simulink model "Plant"  (R2015b)
settings: Solver=ode45  StartTime=0.0  StopTime=1200  RelTol=1e-3
libraries: simulink x2, aerolibanimutils x1
settings Model: Creator=jruesch  LastModifiedBy=jruesch
settings DataIOCC: MaxDataPoints=1  SaveFinalState=on  SaveCompleteFinalSimState=on  SaveFormat=Array  SaveOutput=off  SignalLogging=off  DSMLogging=off  VisualizeSimOutput=off  SaveTime=off
settings HardwareCC: ProdBitPerPointer=32  ProdLargestAtomicFloat=None  ProdIntDivRoundTo=Undefined  ProdEndianess=Unspecified  ProdWordSize=32  ProdHWDeviceType=32-bit Generic
settings GRTTargetCC: GeneratePreprocessorConditionals=Disable all
settings ConfigComp: CovModelRefEnable=Off

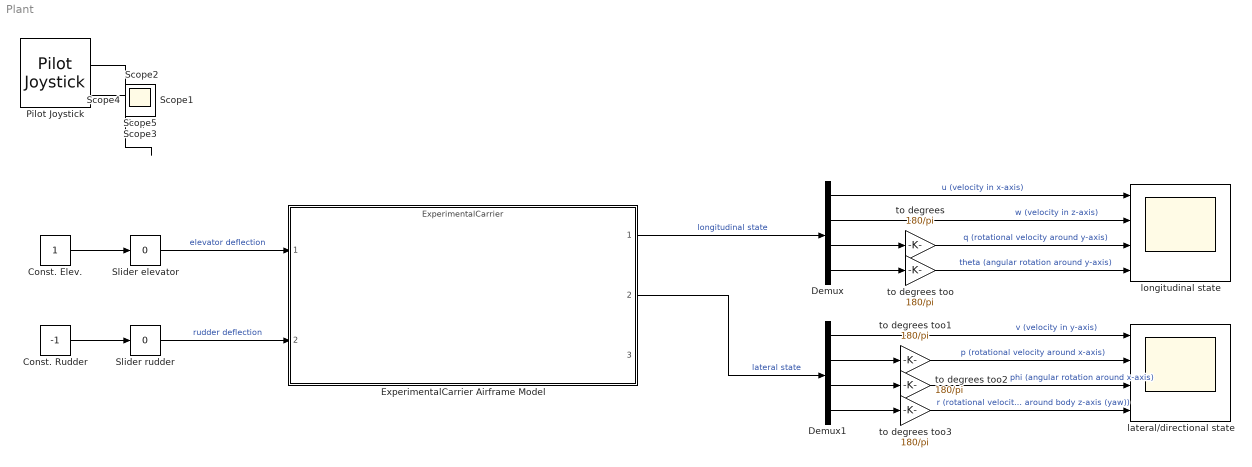
== system Plant ==
  Const. Elev. : Constant
  Const. Rudder : Constant  Value=-1
  Demux : Demux
  Demux1 : Demux
  ExperimentalCarrier Airframe Model : ModelReference  ModelNameDialog=ExperimentalCarrier.slx  SimulationMode=Normal  ModelReferenceVersion=1.534  CopyOfModelName=ExperimentalCarrier.slx
      mask Display: image(imread('../../figures/Airframe01.png'))
  Pilot Joystick : aerolibanimutils/Pilot Joystick  JoystickID=None  OutputConfiguration=FourAxis  SampleTime=1/30
  Slider rudder : simulink/Math Operations/Slider Gain  low=-0.2  gain=0  high=0.2
  Slider elevator : simulink/Math Operations/Slider Gain  low=-0.2  gain=0  high=0.2
  lateral/directional state : Scope  NumInputPorts=4
  longitudinal state : Scope  NumInputPorts=4
  to degrees : Gain  Gain=180/pi
  to degrees too{,1..3} (4 alike) : Gain  Gain=180/pi
  Scope{,1..5} (6 alike) : Scope
  wires:
  Pilot Joystick/4 -> ?
  Pilot Joystick/2 -> ?
  Slider rudder/1 -> ExperimentalCarrier Airframe Model/2  "rudder deflection"
  Slider elevator/1 -> ExperimentalCarrier Airframe Model/1  "elevator deflection"
  ExperimentalCarrier Airframe Model/1 -> Demux/1  "longitudinal state"
  ExperimentalCarrier Airframe Model/2 -> Demux1/1  "lateral state"
  Demux/1 -> longitudinal state/1  "u (velocity in x-axis)"
  Demux/2 -> longitudinal state/2  "w (velocity in z-axis)"
  Demux/3 -> to degrees/1
  Demux/4 -> to degrees too/1
  Demux1/1 -> lateral/directional state/1  "v (velocity in y-axis)"
  Demux1/2 -> to degrees too1/1
  Demux1/3 -> to degrees too2/1
  Demux1/4 -> to degrees too3/1
  to degrees/1 -> longitudinal state/3  "q (rotational velocity around y-axis)"
  to degrees too/1 -> longitudinal state/4  "theta (angular rotation around y-axis)"
  to degrees too1/1 -> lateral/directional state/2  "p (rotational velocity around x-axis)"
  to degrees too2/1 -> lateral/directional state/3  "phi (angular rotation around x-axis)"
  to degrees too3/1 -> lateral/directional state/4  "r (rotational velocity around body z-axis (yaw))"
  Const. Elev./1 -> Slider elevator/1
  Const. Rudder/1 -> Slider rudder/1
